simulink model "model"  (R2023a)
settings: Solver=VariableStepAuto  StartTime=0.0  StopTime=10.0  RelTol=1e-3
undefined symbols (not defined in the file or in its folder): g, m
libraries: shared6dof x1
settings Model: Creator=timme  LastModifiedBy=timme

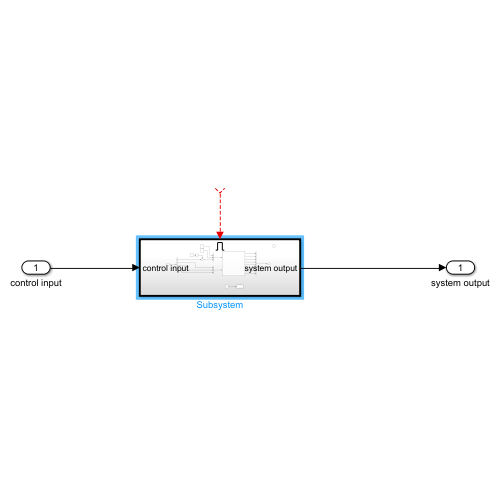
[thumbnail: Simulink's stored preview of the top-level diagram]
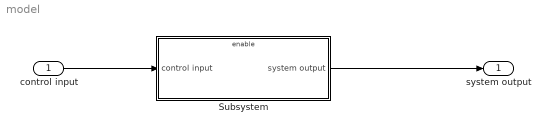
== system model ==
  control input : Inport
  Subsystem : Subsystem
  system output : Outport
  wires:
  control input/1 -> Subsystem/1(control input)
  Subsystem/1(system output) -> system output/1
  ? -> Subsystem/Enable

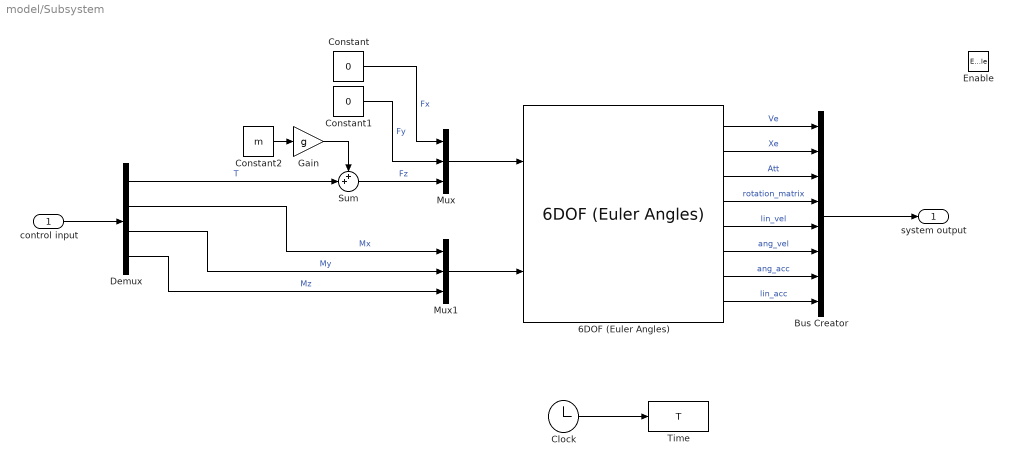
== system model/Subsystem ==
  control input : Inport
  Enable : EnablePort
  6DOF (Euler Angles) : shared6dof/6DOF (Euler Angles)  units=Metric (MKS)  mtype=Fixed  rep=Euler Angles  xme_0=[0 0 0]  Vm_0=[0 0 0]  eul_0=[0 0 0]  pm_0=[0 0 0]  mass_0=m  mass_e=0.5  mass_f=2.0  inertia=I  inertia_e=eye(3)  inertia_f=2*eye(3)  k_quat=1.0  vre_flag=on  abi_flag=off  aMode=0  xme_statename=''  Vm_statename=''  eul_statename=''  quat_statename=''  pm_statename=''  mass_statename=''
  Bus Creator : BusCreator  Inputs=8
  Clock : Clock
  Constant : Constant  Value=0
  Constant1 : Constant  Value=0
  Constant2 : Constant  Value=m
  Demux : Demux
  Gain : Gain  Gain=g
  Mux : Mux  Inputs=3
  Mux1 : Mux  Inputs=3
  Sum : Sum  Inputs=++|
  Time : ToWorkspace  VariableName=T  SampleTime=-1
      settings: Decimation=100
  system output : Outport
  wires:
  Gain/1 -> Sum/1
  Constant2/1 -> Gain/1
  Demux/2 -> Mux1/1  "Mx"
  Clock/1 -> Time/1
  Constant/1 -> Mux/1  "Fx"
  Demux/1 -> Sum/2  "T"
  6DOF (Euler Angles)/2 -> Bus Creator/2  "Xe"
  6DOF (Euler Angles)/8 -> Bus Creator/8  "lin_acc"
  6DOF (Euler Angles)/3 -> Bus Creator/3  "Att"
  Mux1/1 -> 6DOF (Euler Angles)/2
  6DOF (Euler Angles)/7 -> Bus Creator/7  "ang_acc"
  6DOF (Euler Angles)/4 -> Bus Creator/4  "rotation_matrix"
  6DOF (Euler Angles)/1 -> Bus Creator/1  "Ve"
  Bus Creator/1 -> system output/1
  6DOF (Euler Angles)/5 -> Bus Creator/5  "lin_vel"
  6DOF (Euler Angles)/6 -> Bus Creator/6  "ang_vel"
  Demux/4 -> Mux1/3  "Mz"
  Sum/1 -> Mux/3  "Fz"
  Mux/1 -> 6DOF (Euler Angles)/1
  Demux/3 -> Mux1/2  "My"
  control input/1 -> Demux/1
  Constant1/1 -> Mux/2  "Fy"
